simulink model "Recover_Sim"  (R2019b)
settings: Solver=VariableStepAuto  StartTime=0.0  StopTime=10000  RelTol=1e-3
undefined symbols (not defined in the file or in its folder): HDBK, MIL
libraries: simulink x2, dspsrcs4 x2, aerolibatmos2 x1
settings Model: Creator=j90xb  LastModifiedBy=j90xb

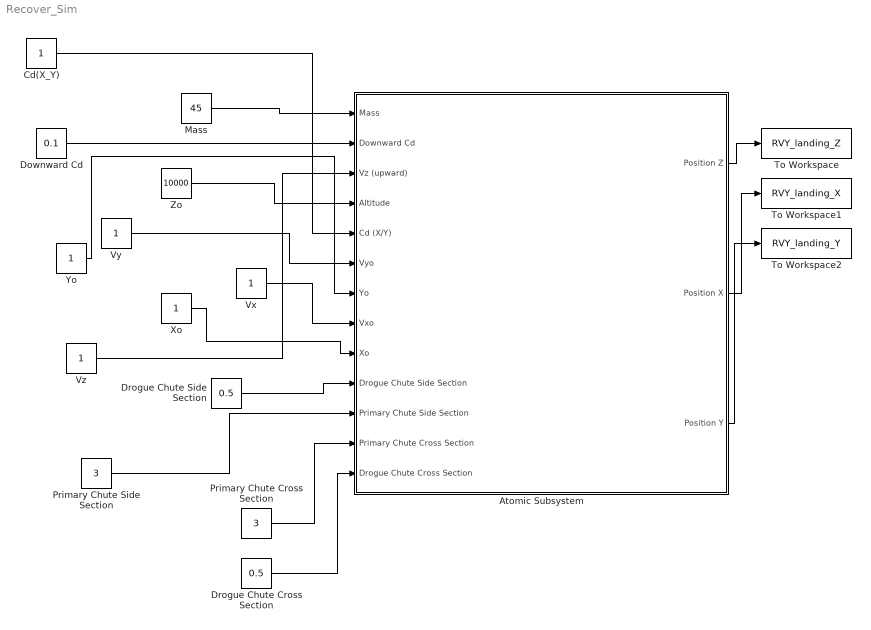
== system Recover_Sim ==
  Atomic Subsystem : Subsystem  TreatAsAtomicUnit=on
  Cd(X_Y) : Constant
  Downward Cd : Constant  Value=0.1
  Drogue Chute Cross Section : Constant  Value=0.5
  Drogue Chute Side Section : Constant  Value=0.5
  Mass : Constant  Value=45
  Primary Chute Cross Section : Constant  Value=3
  Primary Chute Side Section : Constant  Value=3
  To Workspace : ToWorkspace  VariableName=RVY_landing_Z  SampleTime=-1
  To Workspace1 : ToWorkspace  VariableName=RVY_landing_X  SampleTime=-1
  To Workspace2 : ToWorkspace  VariableName=RVY_landing_Y  SampleTime=-1
  Vx : Constant
  Vy : Constant
  Vz : Constant
  Xo : Constant
  Yo : Constant
  Zo : Constant  Value=10000
  wires:
  Atomic Subsystem/1(Position Z) -> To Workspace/1
  Atomic Subsystem/2(Position X) -> To Workspace1/1
  Atomic Subsystem/3(Position Y) -> To Workspace2/1
  Zo/1 -> Atomic Subsystem/4(Altitude)
  Yo/1 -> Atomic Subsystem/7(Yo)
  Xo/1 -> Atomic Subsystem/9(Xo)
  Vy/1 -> Atomic Subsystem/6(Vyo)
  Vx/1 -> Atomic Subsystem/8(Vxo)
  Cd(X_Y)/1 -> Atomic Subsystem/5(Cd (X/Y))
  Mass/1 -> Atomic Subsystem/1(Mass)
  Vz/1 -> Atomic Subsystem/3(Vz (upward))
  Downward Cd/1 -> Atomic Subsystem/2(Downward Cd)
  Drogue Chute Side Section/1 -> Atomic Subsystem/10(Drogue Chute Side Section)
  Primary Chute Side Section/1 -> Atomic Subsystem/11(Primary Chute Side Section)
  Primary Chute Cross Section/1 -> Atomic Subsystem/12(Primary Chute Cross Section)
  Drogue Chute Cross Section/1 -> Atomic Subsystem/13(Drogue Chute Cross Section)

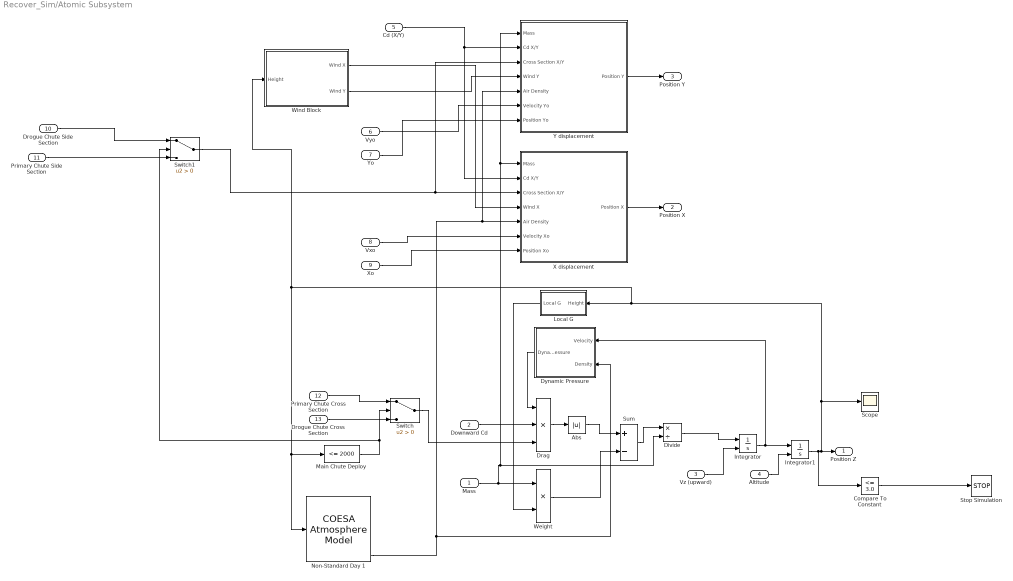
== system Recover_Sim/Atomic Subsystem ==
  Mass : Inport
  Downward Cd : Inport  Port=2
  Vz (upward) : Inport  Port=3
  Altitude : Inport  Port=4
  Cd (X/Y) : Inport  Port=5
  Vyo : Inport  Port=6
  Yo : Inport  Port=7
  Vxo : Inport  Port=8
  Xo : Inport  Port=9
  Drogue Chute Side Section : Inport  Port=10
  Primary Chute Side Section : Inport  Port=11
  Primary Chute Cross Section : Inport  Port=12
  Drogue Chute Cross Section : Inport  Port=13
  Abs : Abs
  Compare To Constant : simulink/Logic and Bit Operations/Compare To Constant  relop=<=  const=3.0  OutDataTypeStr=boolean
  Divide : Product  Inputs=*/
  Drag : Product  Inputs=3
  Dynamic Pressure : Subsystem  TreatAsAtomicUnit=on
  Integrator : Integrator  InitialConditionSource=external
  Integrator1 : Integrator  InitialConditionSource=external
  Local G : Subsystem
  Main Chute Deploy : simulink/Logic and Bit Operations/Compare To Constant  relop=<=  const=2000  OutDataTypeStr=uint8
  Non-Standard Day 1 : aerolibatmos2/COESA Atmosphere Model  units=Metric (MKS)  spec=MIL-HDBK-310  model=Profile  profile_var=High temperature  profile_percent=1%  profile_alt=5 km (16404 ft)  envelope_var=High temperature  envelope_percent=1%  action=Warning
  Scope : Scope
  Stop Simulation : Stop
  Sum : Sum  Inputs=+-
  Switch : Switch  Criteria=u2 > Threshold
  Switch1 : Switch  Criteria=u2 > Threshold
  Weight : Product
  Wind Block : Subsystem  TreatAsAtomicUnit=on
  X displacement : Subsystem  TreatAsAtomicUnit=on
  Y displacement : Subsystem  TreatAsAtomicUnit=on
  Position Z : Outport
  Position X : Outport  Port=2
  Position Y : Outport  Port=3
  wires:
  Drag/1 -> Abs/1
  Switch/1 -> Drag/3
  Sum/1 -> Divide/1
  Vz (upward)/1 -> Integrator/2
  Altitude/1 -> Integrator1/2
  Yo/1 -> Y displacement/7(Position Yo)
  Vyo/1 -> Y displacement/6(Velocity Yo)
  Y displacement/1(Position Y) -> Position Y/1
  Wind Block/2(Wind Y) -> Y displacement/4(Wind Y)
  Switch1/1 -> Y displacement/3(Cross Section X/Y), X displacement/3(Cross Section X/Y)
  Wind Block/1(Wind X) -> X displacement/4(Wind X)
  Integrator1/1 -> Compare To Constant/1, Scope/1, Non-Standard Day 1/1, Main Chute Deploy/1, Wind Block/1(Height), Local G/1(Height), Position Z/1
  Divide/1 -> Integrator/1
  Integrator/1 -> Dynamic Pressure/1("Velocity "), Integrator1/1
  Mass/1 -> X displacement/1(Mass), Y displacement/1(Mass), Divide/2, Weight/1
  Main Chute Deploy/1 -> Switch1/2, Switch/2
  Non-Standard Day 1/4 -> Y displacement/5(Air Density), X displacement/5(Air Density), Dynamic Pressure/2(Density)
  Cd (X/Y)/1 -> X displacement/2(Cd X/Y), Y displacement/2(Cd X/Y)
  Downward Cd/1 -> Drag/2
  Weight/1 -> Sum/2
  Dynamic Pressure/1(Dynamic Pressure) -> Drag/1
  X displacement/1(Position X) -> Position X/1
  Xo/1 -> X displacement/7(Position Xo)
  Local G/1(Local G) -> Weight/2
  Vxo/1 -> X displacement/6(Velocity Xo)
  Compare To Constant/1 -> Stop Simulation/1
  Abs/1 -> Sum/1
  Drogue Chute Side Section/1 -> Switch1/1
  Primary Chute Side Section/1 -> Switch1/3
  Primary Chute Cross Section/1 -> Switch/1
  Drogue Chute Cross Section/1 -> Switch/3

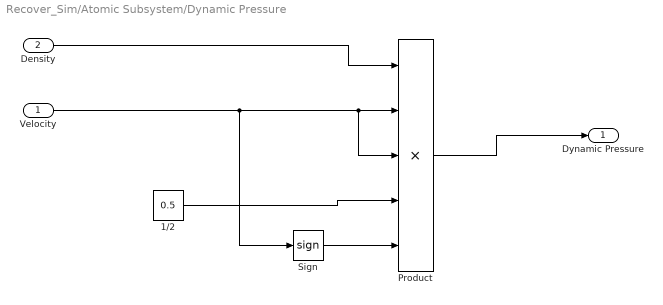
== system Recover_Sim/Atomic Subsystem/Dynamic Pressure ==
  "Velocity " : Inport
  Density : Inport  Port=2
  1/2 : Constant  Value=0.5
  Product : Product  Inputs=5
  Sign : Signum
  Dynamic Pressure : Outport
  wires:
  "Velocity "/1 -> Sign/1, Product/2, Product/3
  Density/1 -> Product/1
  Product/1 -> Dynamic Pressure/1
  1/2/1 -> Product/4
  Sign/1 -> Product/5

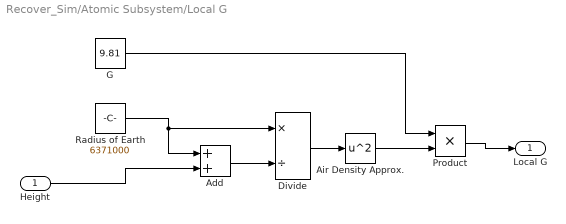
== system Recover_Sim/Atomic Subsystem/Local G ==
  Height : Inport
  Add : Sum
  Air Density Approx. : Math  Operator=square  OutMin=0  OutMax=10000  SaturateOnIntegerOverflow=on
  Divide : Product  Inputs=*/
  G : Constant  Value=9.81
  Product : Product
  Radius of Earth : Constant  Value=6371000
  Local G : Outport  VectorParamsAs1DForOutWhenUnconnected=off
  wires:
  Radius of Earth/1 -> Divide/1, Add/1
  Height/1 -> Add/2
  Add/1 -> Divide/2
  Divide/1 -> Air Density Approx./1
  Air Density Approx./1 -> Product/2
  Product/1 -> Local G/1
  G/1 -> Product/1

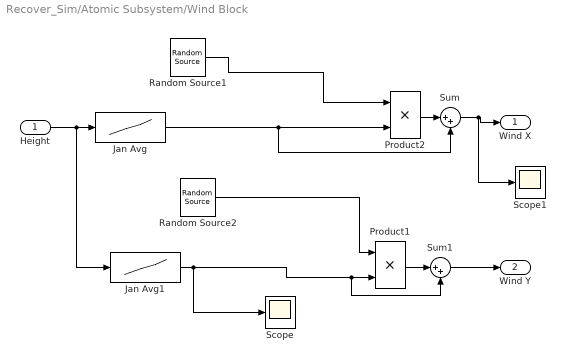
== system Recover_Sim/Atomic Subsystem/Wind Block ==
  Height : Inport
  Jan Avg : Lookup_n-D  NumberOfTableDimensions=1  BreakpointsForDimension1=[0,5000,10000,15000,20000,24000,100000]  IndexSearchMethod=Linear search  Table=[2,17,30,22,5,2,0]  InterpMethod=Cubic spline  ExtrapMethod=Clip  UseLastTableValue=on  InternalRulePriority=Speed  RndMeth=Simplest  InputSameDT=on
  Jan Avg1 : Lookup_n-D  NumberOfTableDimensions=1  BreakpointsForDimension1=[0,5000,10000,15000,20000,24000,100000]  Table=[2,17,30,22,5,2,0]  InterpMethod=Cubic spline  ExtrapMethod=Clip  UseLastTableValue=on  InternalRulePriority=Speed  RndMeth=Simplest  InputSameDT=on
  Product1 : Product
  Product2 : Product
  Random Source1 : dspsrcs4/Random Source  SrcType=Gaussian  NormMethod=Ziggurat  CltLength=12  MinVal=0  MaxVal=1  MeanVal=0  VarVal=0.1  RepMode=Not repeatable  rawSeed=1  IsInherit=off  SampMode=Discrete  SampTime=50000  SampFrame=1  DataType=Double  OutComplex=Real  OutputFrames=off
  Random Source2 : dspsrcs4/Random Source  SrcType=Gaussian  NormMethod=Ziggurat  CltLength=12  MinVal=0  MaxVal=1  MeanVal=0  VarVal=0.1  RepMode=Not repeatable  rawSeed=1  IsInherit=off  SampMode=Discrete  SampTime=50000  SampFrame=1  DataType=Double  OutComplex=Real  OutputFrames=off
  Scope : Scope
  Scope1 : Scope
  Sum : Sum  Inputs=|++
  Sum1 : Sum  Inputs=|++
  Wind X : Outport
  Wind Y : Outport  Port=2
  wires:
  Height/1 -> Jan Avg1/1, Jan Avg/1
  Jan Avg/1 -> Sum/2, Product2/2
  Jan Avg1/1 -> Scope/1, Sum1/2, Product1/2
  Random Source1/1 -> Product2/1
  Random Source2/1 -> Product1/1
  Product2/1 -> Sum/1
  Sum/1 -> Scope1/1, Wind X/1
  Product1/1 -> Sum1/1
  Sum1/1 -> Wind Y/1

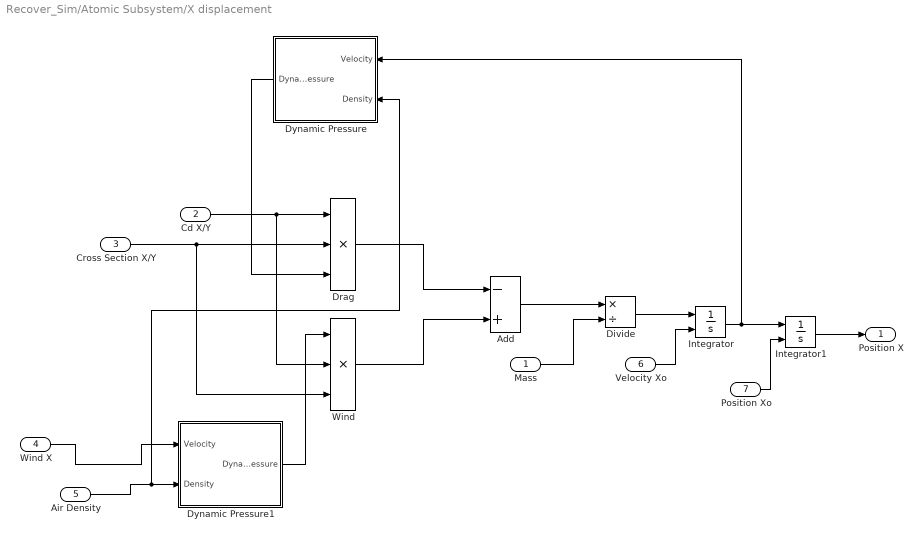
== system Recover_Sim/Atomic Subsystem/X displacement ==
  Mass : Inport
  Cd X/Y : Inport  Port=2
  Cross Section X/Y : Inport  Port=3
  Wind X : Inport  Port=4
  Air Density : Inport  Port=5
  Velocity Xo : Inport  Port=6
  Position Xo : Inport  Port=7
  Add : Sum  Inputs=-+
  Divide : Product  Inputs=*/
  Drag : Product  Inputs=3
  Dynamic Pressure : Subsystem  TreatAsAtomicUnit=on
  Dynamic Pressure1 : Subsystem  TreatAsAtomicUnit=on
  Integrator : Integrator  InitialConditionSource=external
  Integrator1 : Integrator  InitialConditionSource=external
  Wind : Product  Inputs=3
  Position X : Outport
  wires:
  Add/1 -> Divide/1
  Mass/1 -> Divide/2
  Wind/1 -> Add/2
  Drag/1 -> Add/1
  Cd X/Y/1 -> Wind/2, Drag/1
  Cross Section X/Y/1 -> Wind/3, Drag/2
  Dynamic Pressure/1(Dynamic Pressure) -> Drag/3
  Divide/1 -> Integrator/1
  Integrator/1 -> Dynamic Pressure/1("Velocity "), Integrator1/1
  Integrator1/1 -> Position X/1
  Dynamic Pressure1/1(Dynamic Pressure) -> Wind/1
  Air Density/1 -> Dynamic Pressure/2(Density), Dynamic Pressure1/2(Density)
  Velocity Xo/1 -> Integrator/2
  Position Xo/1 -> Integrator1/2
  Wind X/1 -> Dynamic Pressure1/1("Velocity ")

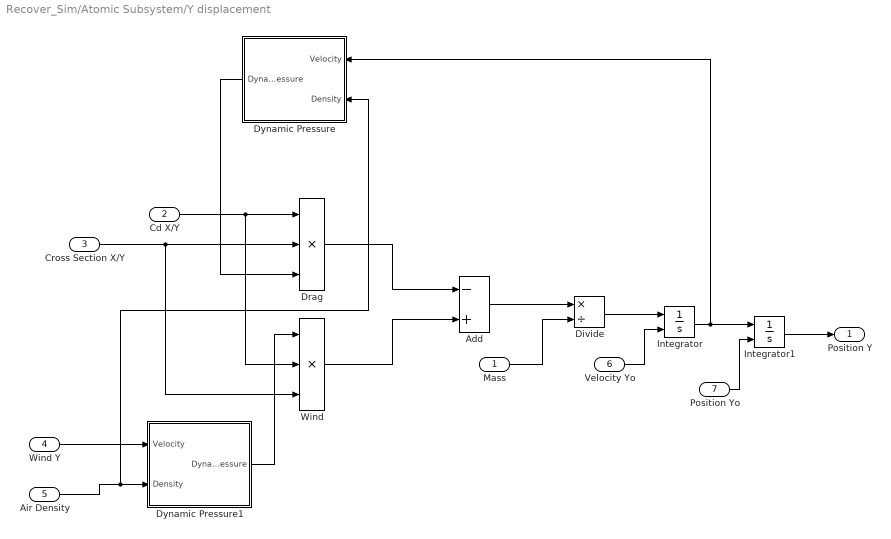
== system Recover_Sim/Atomic Subsystem/Y displacement ==
  Mass : Inport
  Cd X/Y : Inport  Port=2
  Cross Section X/Y : Inport  Port=3
  Wind Y : Inport  Port=4
  Air Density : Inport  Port=5
  Velocity Yo : Inport  Port=6
  Position Yo : Inport  Port=7
  Add : Sum  Inputs=-+
  Divide : Product  Inputs=*/
  Drag : Product  Inputs=3
  Dynamic Pressure : Subsystem  TreatAsAtomicUnit=on
  Dynamic Pressure1 : Subsystem  TreatAsAtomicUnit=on
  Integrator : Integrator  InitialConditionSource=external
  Integrator1 : Integrator  InitialConditionSource=external
  Wind : Product  Inputs=3
  Position Y : Outport
  wires:
  Add/1 -> Divide/1
  Mass/1 -> Divide/2
  Wind/1 -> Add/2
  Drag/1 -> Add/1
  Cd X/Y/1 -> Wind/2, Drag/1
  Cross Section X/Y/1 -> Wind/3, Drag/2
  Dynamic Pressure/1(Dynamic Pressure) -> Drag/3
  Divide/1 -> Integrator/1
  Integrator/1 -> Dynamic Pressure/1("Velocity "), Integrator1/1
  Integrator1/1 -> Position Y/1
  Dynamic Pressure1/1(Dynamic Pressure) -> Wind/1
  Wind Y/1 -> Dynamic Pressure1/1("Velocity ")
  Air Density/1 -> Dynamic Pressure/2(Density), Dynamic Pressure1/2(Density)
  Velocity Yo/1 -> Integrator/2
  Position Yo/1 -> Integrator1/2

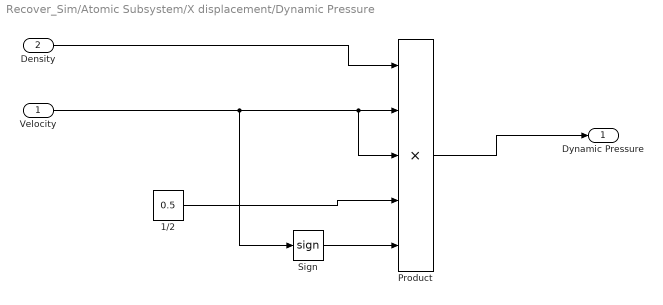
== system Recover_Sim/Atomic Subsystem/X displacement/Dynamic Pressure ==
  "Velocity " : Inport
  Density : Inport  Port=2
  1/2 : Constant  Value=0.5
  Product : Product  Inputs=5
  Sign : Signum
  Dynamic Pressure : Outport
  wires:
  "Velocity "/1 -> Sign/1, Product/2, Product/3
  Density/1 -> Product/1
  Product/1 -> Dynamic Pressure/1
  1/2/1 -> Product/4
  Sign/1 -> Product/5

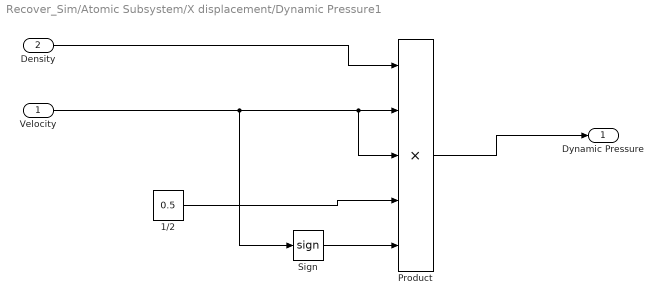
== system Recover_Sim/Atomic Subsystem/X displacement/Dynamic Pressure1 ==
  "Velocity " : Inport
  Density : Inport  Port=2
  1/2 : Constant  Value=0.5
  Product : Product  Inputs=5
  Sign : Signum
  Dynamic Pressure : Outport
  wires:
  "Velocity "/1 -> Sign/1, Product/2, Product/3
  Density/1 -> Product/1
  Product/1 -> Dynamic Pressure/1
  1/2/1 -> Product/4
  Sign/1 -> Product/5

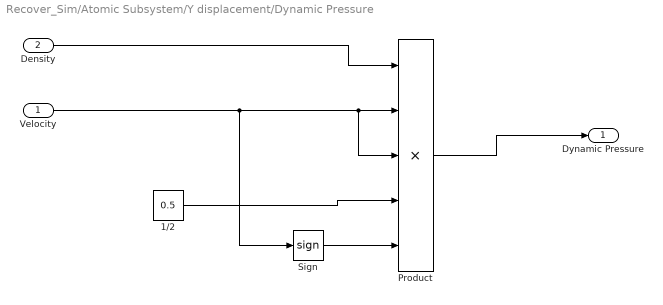
== system Recover_Sim/Atomic Subsystem/Y displacement/Dynamic Pressure ==
  "Velocity " : Inport
  Density : Inport  Port=2
  1/2 : Constant  Value=0.5
  Product : Product  Inputs=5
  Sign : Signum
  Dynamic Pressure : Outport
  wires:
  "Velocity "/1 -> Sign/1, Product/2, Product/3
  Density/1 -> Product/1
  Product/1 -> Dynamic Pressure/1
  1/2/1 -> Product/4
  Sign/1 -> Product/5

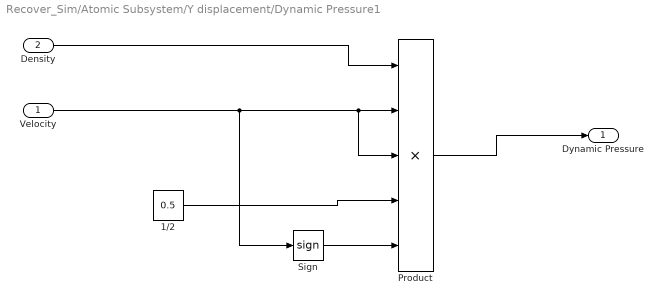
== system Recover_Sim/Atomic Subsystem/Y displacement/Dynamic Pressure1 ==
  "Velocity " : Inport
  Density : Inport  Port=2
  1/2 : Constant  Value=0.5
  Product : Product  Inputs=5
  Sign : Signum
  Dynamic Pressure : Outport
  wires:
  "Velocity "/1 -> Sign/1, Product/2, Product/3
  Density/1 -> Product/1
  Product/1 -> Dynamic Pressure/1
  1/2/1 -> Product/4
  Sign/1 -> Product/5
